simulink model "mass_spring_damper_KF_vs_EKF"  (R2019b)
settings: Solver=FixedStepAuto  StartTime=0.0  StopTime=200  FixedStep=0.01  RelTol=1e-3
values from neighbouring files (symbols this model uses):
  A = [0.969169519504925  -0.246386829627017;  0.049277365925403  0.993808202467626]    [DMDc_MW.m]    (also in DMDc_param_sweep.m = real(A); EKF_msd_estimator.m = [0, 1; -k/m, -b/m]; HAVOK.m = AB(:,1:q*m); HAVOK_param_sweep.m = real(A))
  B = [0.049277365925403; 0.001238359506475]    [DMDc_MW.m]    (also in DMDc_param_sweep.m = AB(:,(q*m+1):end); EKF_estimator.m = zeros(nx,1); EKF_msd_estimator.m = [0; 1/m]; HAVOK.m = AB(:,(q*m+1):end))
  b = c(2)    [EKF_estimator.m]    (also in EKF_msd_estimator.m = 0.01; KF_estimator.m = 0.01; Linear_regression_parameter_estimator.m = 0.5; cart_pend_EKF_script.m)
  C = [0 1]    [DMDc_MW.m]    (also in EKF_estimator.m = eye(6); EKF_msd_estimator.m = [1, 0]; KF_estimator.m = [1, 0]; LS.m)
  D = 0    [DMDc_MW.m]    (also in DMDc_param_sweep.m = (q-1)*Ts; EKF_estimator.m = m*L*L*(M+m*(1-Cx^2)); EKF_msd_estimator.m; HAVOK.m = 3.99)
  f = f_data(k)    [DMDc_MW.m]    (also in EKF_estimator.m = @cartpend; EKF_msd_estimator.m = @msd; HAVOK.m = @nl_msd; LS.m = out.f.Data')
  g = -9.81    [EKF_estimator.m]    (also in cart_pend_EKF_script.m; cart_pend_EKF_setup.m; cart_pend_NLLS.m = 9.81; floating_pendulum_2D.m = -abs(g))
  k = c(3)    [EKF_estimator.m]    (also in EKF_msd_estimator.m = 5; HAVOK.m = 1.1; KF_estimator.m = 5; Linear_regression_parameter_estimator.m = 5)
  m = size(y_data,1)    [DMDc_param_sweep.m]    (also in EKF_estimator.m = numel(f_x); EKF_msd_estimator.m = numel(f_x); HAVOK.m = 1; HAVOK_param_sweep.m)
  P0 = 0.01*eye(nx)    [EKF_estimator.m]    (also in EKF_msd_estimator.m = [0.1, 0.1; 0.1, 0.1]; KF_estimator.m = [0, 0; 0, 0]; cart_pend_EKF_script.m; cart_pend_EKF_setup.m = 0.1*eye(nx))
  Q = 0.01*eye(nx)    [EKF_estimator.m]    (also in EKF_msd_estimator.m = 0.00000001*eye(nx); KF_estimator.m = B*(sigma_a^2)*B'; cart_pend_EKF_script.m; cart_pend_EKF_setup.m = diag([0; 0.00001; 0; 0.00001; 0.00001; 0.00001; 0.00001; 0.0)
  R = 0.0001*eye(ny)    [EKF_estimator.m]    (also in EKF_msd_estimator.m = 0.01*eye(ny); KF_estimator.m = 0.01; cart_pend_EKF_script.m; cart_pend_EKF_setup.m = 0.001*eye(ny))
  Ts = 0.05    [DMDc_MW.m]    (also in DMDc_param_sweep.m = t(2)-t(1); EKF_msd_estimator.m = 0.01; HAVOK.m = t(2)-t(1); HAVOK_param_sweep.m = t(2)-t(1))
  u0 = 0    [cart_pend_EKF_setup.m]    (also in mass_spring_damper_EKF_param_script.m; mass_spring_damper_EKF_script.m; mass_spring_damper_EKF_setup.m)
  x0 = [0; 0; 0; 0; 0; 1]    [EKF_estimator.m]    (also in EKF_msd_estimator.m = [0; 0]; HAVOK.m = [0.5; 0]; KF_estimator.m = [0; 0]; Linear_regression_state_estimator.m = [0;0;0;0])
settings Model: Creator=Murray  LastModifiedBy=Murray

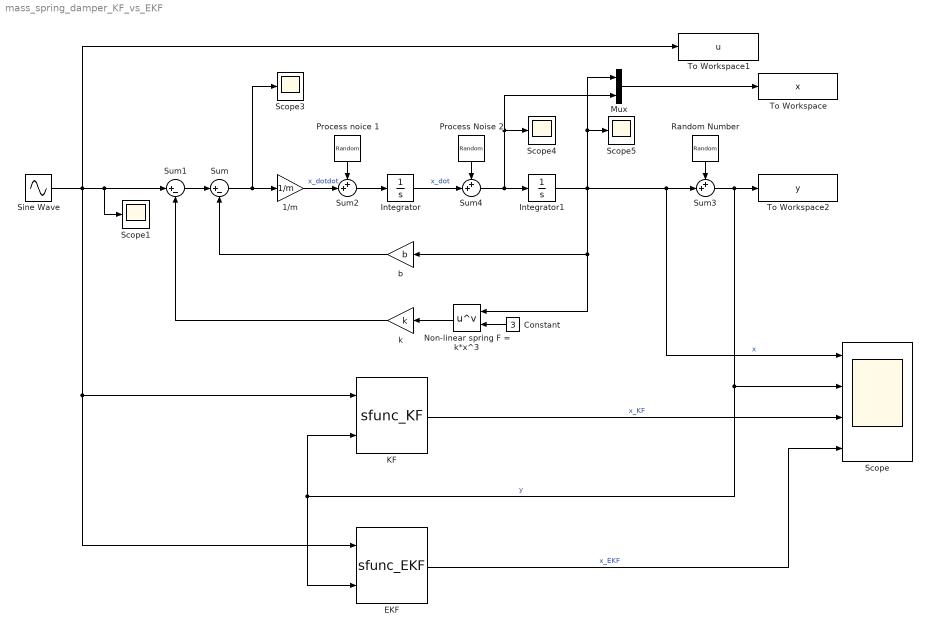
== system mass_spring_damper_KF_vs_EKF ==
  1/m : Gain  Gain=1/m
  Constant : Constant  Value=3
  EKF : M-S-Function  FunctionName=sfunc_EKF  Parameters=Ts,f,g,Q,R,x0,P0,u0
      mask Display:
      | port_label('input', 1, 'u')
      | port_label('input', 2, 'y')
      | port_label('output', 1, 'x_hat')
  Integrator : Integrator
  Integrator1 : Integrator
  KF : M-S-Function  FunctionName=sfunc_KF  Parameters=A,B,C,D,Ts,Q,R,x0,P0
      mask Display:
      | port_label('input', 1, 'u')
      | port_label('input', 2, 'y')
      | port_label('output', 1, 'x_hat')
  Mux : Mux  Inputs=2
  Non-linear spring F = k*x^3 : Math  Operator=pow  SignedPower=off  SaturateOnIntegerOverflow=on
  Process Noise 2 : RandomNumber  Variance=0.0001  SampleTime=0.01
  Process noice 1 : RandomNumber  Variance=0.0001  SampleTime=0.01
  Random Number : RandomNumber  Variance=R  SampleTime=0.01
  Scope : Scope  NumInputPorts=4
  Scope{1,3..5} (4 alike) : Scope
  Sine Wave : Sin  Bias=2  Frequency=pi/4  SampleTime=0
  Sum : Sum  Inputs=|+-
  Sum1 : Sum  Inputs=|+-
  Sum2 : Sum  Inputs=++|
  Sum3 : Sum  Inputs=++|
  Sum4 : Sum  Inputs=++|
  To Workspace : ToWorkspace  VariableName=x  SaveFormat=Timeseries  SampleTime=-1
  To Workspace1 : ToWorkspace  VariableName=u  SaveFormat=Timeseries  SampleTime=-1
  To Workspace2 : ToWorkspace  VariableName=y  SaveFormat=Timeseries  SampleTime=-1
  b : Gain  Gain=b
  k : Gain  Gain=k
  wires:
  Sum/1 -> Scope3/1, 1/m/1
  b/1 -> Sum/2
  Sum1/1 -> Sum/1
  Integrator1/1 -> Scope5/1, Mux/1, Non-linear spring F = k*x^3/1, b/1, Scope/1, Sum3/2  "x"
  Sine Wave/1 -> Scope1/1, Sum1/1, EKF/1, KF/1, To Workspace1/1
  k/1 -> Sum1/2
  Random Number/1 -> Sum3/1
  Mux/1 -> To Workspace/1
  Sum3/1 -> To Workspace2/1, EKF/2, KF/2, Scope/2  "y"
  KF/1 -> Scope/3  "x_KF"
  EKF/1 -> Scope/4  "x_EKF"
  Process noice 1/1 -> Sum2/1
  Process Noise 2/1 -> Sum4/1
  Integrator/1 -> Sum4/2  "x_dot"
  Sum4/1 -> Scope4/1, Mux/2, Integrator1/1
  Sum2/1 -> Integrator/1
  1/m/1 -> Sum2/2  "x_dotdot"
  Constant/1 -> Non-linear spring F = k*x^3/2
  Non-linear spring F = k*x^3/1 -> k/1
